simulink model "LoadFlow58BusNetwork_2024"  (R2024a)
settings: Solver=FixedStepDiscrete  StartTime=0.0  StopTime=4.5  FixedStep=75e-6  RelTol=1e-3  EnableMultiTasking=on
undefined symbols (not defined in the file): D1, D11, Delta
libraries: spsSeriesRLCBranchLib x41, spsLoadFlowBusLib x29, spsDistributedParametersLineLib x19, spsThreePhaseSeriesRLCLoadLib x15, spsThreePhaseTransformerTwoWindingsLib x13, spsThreePhaseParallelRLCLoadLib x11, spsThreePhaseVIMeasurementLib x11, spsSynchronousMachinepuStandardLib x7, spsExcitationSystemLib x7, spsHydraulicTurbineandGovernorLib x7, spsGenericPowerSystemStabilizerLib x7, spsMultiBandPowerSystemStabilizerLib x7
(part 2 of 5)

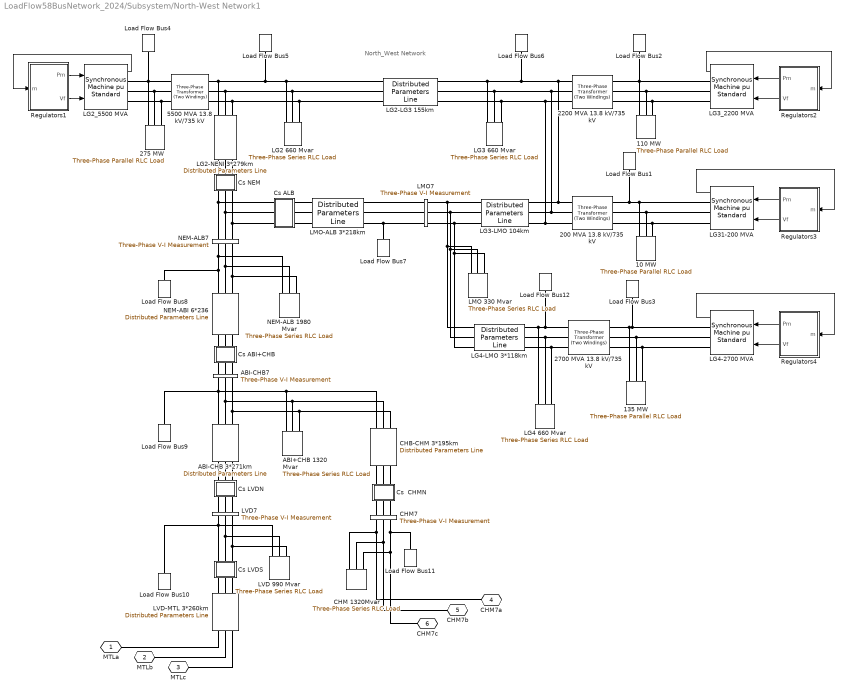
== system LoadFlow58BusNetwork_2024/Subsystem/North-West Network1 ==
  note: North_West Network
  10 MW : spsThreePhaseParallelRLCLoadLib/Three-Phase Parallel RLC Load  LConnTagsString=A|B|C  Configuration=Y (grounded)  NominalVoltage=(13800)*1  Vabc=[1e3 1e3 1e3]  Vabcp=[1e3 1e3 1e3]  NominalFrequency=60  UnbalancedPower=off  ActivePower=10000000  InductivePower=0  CapacitivePower=0  Pabc=[10e3 9e3 11e3]  QLabc=[100 90 110]  QCabc=[100 90 110]  Pabcp=[10e3 9e3 11e3]  QLabcp=[100 90 110]  QCabcp=[100 90 110]  Measurements=None  LoadType=constant PQ
  110 MW : spsThreePhaseParallelRLCLoadLib/Three-Phase Parallel RLC Load  LConnTagsString=A|B|C  Configuration=Y (grounded)  NominalVoltage=(13800)*1  Vabc=[1e3 1e3 1e3]  Vabcp=[1e3 1e3 1e3]  NominalFrequency=60  UnbalancedPower=off  ActivePower=110000000  InductivePower=0  CapacitivePower=0  Pabc=[10e3 9e3 11e3]  QLabc=[100 90 110]  QCabc=[100 90 110]  Pabcp=[10e3 9e3 11e3]  QLabcp=[100 90 110]  QCabcp=[100 90 110]  Measurements=None  LoadType=constant PQ
  135 MW : spsThreePhaseParallelRLCLoadLib/Three-Phase Parallel RLC Load  LConnTagsString=A|B|C  Configuration=Y (grounded)  NominalVoltage=(13800)*1  Vabc=[1e3 1e3 1e3]  Vabcp=[1e3 1e3 1e3]  NominalFrequency=60  UnbalancedPower=off  ActivePower=135000000  InductivePower=0  CapacitivePower=0  Pabc=[10e3 9e3 11e3]  QLabc=[100 90 110]  QCabc=[100 90 110]  Pabcp=[10e3 9e3 11e3]  QLabcp=[100 90 110]  QCabcp=[100 90 110]  Measurements=None  LoadType=constant PQ
  200 MVA 13.8 kV/735 kV : spsThreePhaseTransformerTwoWindingsLib/Three-Phase Transformer (Two Windings)  Winding1Connection=Delta (D1)  Winding2Connection=Yg  CoreType=Three single-phase transformers  SetSaturation=off  Hysteresis=off  DataFile='basic_model'  SetInitialFlux=off  Measurements=None  UNITS=pu  NominalPower=[ 200e6 60 ]  Winding1="[ 13.8e3 0.002  0.0]"  Winding2=[ 735e3 0.002 0.12]  Rm=500  Lm=500  L0=0.5  Saturation="[ 0,0  ;  0.005,1.2  ;  1.0,1.4 ]"  InitialFluxes=[ 0.8 , -0.8 , 0.7 ]  BreakLoop=off  DiscreteSolver=Trapezoidal iterative  DataType=off  TransfoNumber=0
  2200 MVA 13.8 kV/735 kV : spsThreePhaseTransformerTwoWindingsLib/Three-Phase Transformer (Two Windings)  Winding1Connection=Delta (D1)  Winding2Connection=Yg  CoreType=Three single-phase transformers  SetSaturation=off  Hysteresis=off  DataFile='basic_model'  SetInitialFlux=off  Measurements=None  UNITS=pu  NominalPower=[ 2200e6 60 ]  Winding1="[ 13.8e3 0.002  0.0]"  Winding2=[ 735e3 0.002 0.12]  Rm=500  Lm=500  L0=0.5  Saturation="[ 0,0  ;  0.005,1.2  ;  1.0,1.4 ]"  InitialFluxes=[ 0.8 , -0.8 , 0.7 ]  BreakLoop=off  DiscreteSolver=Trapezoidal iterative  DataType=off  TransfoNumber=0
  2700 MVA 13.8 kV/735 kV : spsThreePhaseTransformerTwoWindingsLib/Three-Phase Transformer (Two Windings)  Winding1Connection=Delta (D1)  Winding2Connection=Yg  CoreType=Three single-phase transformers  SetSaturation=off  Hysteresis=off  DataFile='basic_model'  SetInitialFlux=off  Measurements=None  UNITS=pu  NominalPower=[ 2700e6 60 ]  Winding1="[ 13.8e3 0.002  0.0]"  Winding2=[ 735e3 0.002 0.12]  Rm=500  Lm=500  L0=0.5  Saturation="[ 0,0  ;  0.005,1.2  ;  1.0,1.4 ]"  InitialFluxes=[ 0.8 , -0.8 , 0.7 ]  BreakLoop=off  DiscreteSolver=Trapezoidal iterative  DataType=off  TransfoNumber=0
  275 MW : spsThreePhaseParallelRLCLoadLib/Three-Phase Parallel RLC Load  LConnTagsString=A|B|C  Configuration=Y (grounded)  NominalVoltage=(13800)*1  Vabc=[1e3 1e3 1e3]  Vabcp=[1e3 1e3 1e3]  NominalFrequency=60  UnbalancedPower=off  ActivePower=275000000  InductivePower=0  CapacitivePower=0  Pabc=[10e3 9e3 11e3]  QLabc=[100 90 110]  QCabc=[100 90 110]  Pabcp=[10e3 9e3 11e3]  QLabcp=[100 90 110]  QCabcp=[100 90 110]  Measurements=None  LoadType=constant PQ
  5500 MVA 13.8 kV/735 kV : spsThreePhaseTransformerTwoWindingsLib/Three-Phase Transformer (Two Windings)  Winding1Connection=Delta (D1)  Winding2Connection=Yg  CoreType=Three single-phase transformers  SetSaturation=off  Hysteresis=off  DataFile='basic_model'  SetInitialFlux=off  Measurements=None  UNITS=pu  NominalPower=[ 5500e6 60 ]  Winding1="[ 13.8e3 0.002  0.0]"  Winding2=[ 735e3 0.002 0.12]  Rm=500  Lm=500  L0=0.5  Saturation="[ 0,0  ;  0.005,1.2  ;  1.0,1.4 ]"  InitialFluxes=[ 0.8 , -0.8 , 0.7 ]  BreakLoop=off  DiscreteSolver=Trapezoidal iterative  DataType=off  TransfoNumber=0
  ABI+CHB 1320 Mvar : spsThreePhaseSeriesRLCLoadLib/Three-Phase Series RLC Load  LConnTagsString=A|B|C  Configuration=Y (grounded)  NominalVoltage=735e3  Vabc=[1e3 1e3 1e3]  Vabcp=[1e3 1e3 1e3]  NominalFrequency=60  UnbalancedPower=off  ActivePower=4400000  InductivePower=1320e6  CapacitivePower=0  Pabc=[10e3 9e3 11e3]  QLabc=[100 90 110]  QCabc=[100 90 110]  Pabcp=[10e3 9e3 11e3]  QLabcp=[100 90 110]  QCabcp=[100 90 110]  Measurements=None  LoadType=constant Z
  ABI-CHB 3*271km : spsDistributedParametersLineLib/Distributed Parameters Line  Phases=3  Length=271  Frequency=60  Resistance="[0.01273  0.3864]/3"  Inductance="[0.9337e-3  4.1264e-3]/3"  Capacitance=[12.74e-9 7.751e-9]*3  x1=[-0.001575 2.74195871490081e-08 -34814.2579740979 -747194.944177986;-0.0015 2.75338105936338e-08 -13676.7298713989 -747880.497252652;-0.001425 2.76260239313523e-08 7471.73119989829 -747968.20610077;-0.00135 2.76961534482325e-08 28614.2194835957 -747458.000609228;-0.001275 2.77441430838115e-08 49733.83399805 -746350.28862849;-0.0012 2.77699544759089e-08 70813.6920465595 -744645.955646565;-0.001125 2.77735669912929e-08 91836.9427131329 -742346.364081161;-0.00105 2.77549777421738e-08 112786.780332854 -739453.352190591;-0.000975 2.7714201588513e-08 133646.457926072 -735969.232604295;-0.0009 2.76512711261439e-08 154399.300585684 -731896.790474162;-0.000825 2.75662366607152e-08 175028.718806795 -727239.281248121;-0.00075 2.74591661674775e-08 195518.221748122 -722000.428067784;-0.000675 2.73301452369448e-08 215851.430414513 -716184.418792227;-0.0006 2.7179277006475e-08 236012.090750068 -709795.902650276;-0.000525 2.7006682077823e-08 255984.086631383 -702839.986523989;-0.00045 2.68124984207341e-08 275751.452750533 -695322.230866286;-0.000375 2.65968812626527e-08 295298.387377493 -687248.645256015;-0.0003 2.63600029646359e-08 314609.264991801 -678625.683593984;-0.000225 2.61020528835707e-08 333668.648773357 -669460.238943809;-0.00015 2.58232372208051e-08 352461.302942385 -659759.638021708;-7.5e-05 2.55237788573141e-08 370972.20493868 -649531.635339633]  x2=[-0.001575 6.23609378461212e-08 -284619.341076135 -691578.758256646;-0.0015 6.2553714796313e-08 -264954.255311327 -699348.68385095;-0.001425 6.26964872640005e-08 -245077.369168759 -706559.560807776;-0.00135 6.27891411190576e-08 -225004.571927087 -713205.624862417;-0.001275 6.28316022954102e-08 -204751.909473303 -719281.563252954;-0.0012 6.28238368502436e-08 -184335.571475894 -724782.518967204;-0.001125 6.27658509911358e-08 -163771.878443077 -729704.094625337;-0.00105 6.26576910710955e-08 -143077.268676425 -734042.355995072;-0.000975 6.24994435515077e-08 -122268.28513035 -737793.83513665;-0.0009 6.22912349330185e-08 -101361.562187909 -740955.533175044;-0.000825 6.20332316544116e-08 -80373.8123635385 -743524.922697218;-0.00075 6.17256399595605e-08 -59321.8129433254 -745499.9497725;-0.000675 6.13687057325596e-08 -38222.3925734996 -746879.035594466;-0.0006 6.09627143011688e-08 -17092.4178078727 -747661.07774301;-0.000525 6.05079902087265e-08 4051.22037502704 -747845.451065604;-0.00045 6.00048969547146e-08 25191.6200743447 -747432.008177036;-0.000375 5.94538367041829e-08 46311.8819780197 -746421.079577224;-0.0003 5.8855249966264e-08 67395.122871837 -744813.473387024;-0.000225 5.82096152420376e-08 88424.4891356105 -742610.474702226;-0.00015 5.75174486420237e-08 109383.170215709 -739813.844566273;-7.5e-05 5.67793034736118e-08 130254.412063156 -736425.818562504]  x3=[-0.001575 1.26976511809194e-10 -354.964030660685 -109.750554353959;-0.0015 1.34931646331752e-10 -351.719210477034 -119.741131838097;-0.001425 1.42778918560755e-10 -348.193231338013 -129.635990093544;-0.00135 1.50512055506852e-10 -344.388911857396 -139.427219322008;-0.001275 1.58124875418688e-10 -340.309293149966 -149.106992564654;-0.0012 1.65611292724507e-10 -335.957636400499 -158.667571958857;-0.001125 1.72965322896859e-10 -331.337420256818 -168.101314923731;-0.00105 1.80181087236545e-10 -326.452338049017 -177.400680269492;-0.000975 1.87252817571958e-10 -321.306294837067 -186.558234225766;-0.0009 1.94174860870068e-10 -315.903404289175 -195.566656384037;-0.000825 2.00941683755373e-10 -310.247985393379 -204.418745549465;-0.00075 2.07547876933195e-10 -304.344559005013 -213.107425497413;-0.000675 2.13988159513786e-10 -298.197844232806 -221.625750630071;-0.0006 2.2025738323379e-10 -291.812754666499 -229.966911528663;-0.000525 2.26350536571688e-10 -285.194394448997 -238.12424039679;-0.00045 2.3226274875393e-10 -278.348054196193 -246.091216390567;-0.000375 2.37989293648557e-10 -271.279206767732 -253.861470831284;-0.0003 2.435255935432e-10 -263.993502892093 -261.428792296429;-0.000225 2.48867222804431e-10 -256.496766649477 -268.787131585007;-0.00015 2.54009911415548e-10 -248.794990816134 -275.930606553176;-7.5e-05 2.58949548389962e-10 -240.894332073824 -282.853506816347]  x4=[-0.001575 1.8709121084467e-10 -5971.27343085291 -15054.8004559038;-0.0015 1.83115936519456e-10 -5543.2793985662 -15217.5948036282;-0.001425 1.78994282116356e-10 -5110.85415354329 -15368.2244389036;-0.00135 1.74729542422837e-10 -4674.34336990873 -15506.5689507043;-0.001275 1.70325126606556e-10 -4234.09598770412 -15632.5177485442;-0.0012 1.65784555490128e-10 -3790.46393395078 -15745.9701508815;-0.001125 1.6111145873663e-10 -3343.80184132468 -15846.8354656016;-0.00105 1.56309571948106e-10 -2894.46676466851 -15935.0330625152;-0.000975 1.51382733679383e-10 -2442.81789556749 -16010.4924378129;-0.0009 1.46334882369591e-10 -1989.21627521713 -16073.1532704244;-0.000825 1.41170053193831e-10 -1534.02450581238 -16122.9654702391;-0.00075 1.35892374837522e-10 -1077.60646068905 -16159.8892181466;-0.000675 1.3050606619599e-10 -620.326993448974 -16183.8949978676;-0.0006 1.25015433001952e-10 -162.551646301657 -16194.9636195492;-0.000525 1.19424864383572e-10 295.353642144589 -16193.0862351047;-0.00045 1.13738829355866e-10 753.022829408368 -16178.2643452863;-0.000375 1.07961873248235e-10 1210.09006174395 -16150.509798486;-0.0003 1.02098614071001e-10 1666.18996659918 -16109.8447812639;-0.000225 9.61537388238404e-11 2120.95794468867 -16056.3018006126;-0.00015 9.01319997490654e-11 2574.03046144892 -15989.9236579715;-7.5e-05 8.40382105327568e-11 3025.04533764227 -15910.7634150122]  x5=0.00153261764655846  V1=ones(3,3)  V2=ones(3,3)  I1=ones(3,3)  I2=ones(3,3)  nHarmo=1  Measurements=None  Decoupling=on  VsMag0=[610743.955114576 610743.501375021 610743.958218031]  VrMag0=[610622.360478061 610622.247686743 610622.214003654]  VsAngle0=[1.35232982185966 -118.647645266061 121.352379141747]  VrAngle0=[-18.3496130787512 -138.34962283858 101.650391206841]  IsMag0=[305.299965909112 305.301188713068 305.286778308149]  IrMag0=[13308.3117169381 13308.3164139128 13308.3246262143]  IsAngle0=[-68.7963830004266 171.200626740019 51.2019231191185]  IrAngle0=[-17.6151010152143 -137.615048514484 102.384907722659]
      settings: AttributesFormatString=\n  LibrarySourceBlock=sps_lib/Power Grid Elements/Distributed Parameters Line
  ABI-CHB7 : spsThreePhaseVIMeasurementLib/Three-Phase V-I Measurement  VoltageMeasurement=no  SetLabelV=on  LabelV=Vabc_ABI7  Vpu=on  VpuLL=off  CurrentMeasurement=no  SetLabelI=off  LabelI=A1  Ipu=off  Pbase=100e6  Vbase=500e3  OutputType=Magnitude  PhasorSimulation=off  PSBequivalent=0
  CHB-CHM 3*195km : spsDistributedParametersLineLib/Distributed Parameters Line  Phases=3  Length=195  Frequency=60  Resistance="[0.01273  0.3864]/3"  Inductance="[0.9337e-3  4.1264e-3]/3"  Capacitance=[12.74e-9 7.751e-9]*3  x1=[-0.001125 2.77735669912929e-08 0 0;-0.00105 2.77549777421738e-08 0 0;-0.000975 2.7714201588513e-08 0 0;-0.0009 2.76512711261439e-08 0 0;-0.000825 2.75662366607152e-08 0 0;-0.00075 2.74591661674775e-08 0 0;-0.000675 2.73301452369448e-08 215851.430414513 -716184.418792227;-0.0006 2.7179277006475e-08 236012.090750068 -709795.902650276;-0.000525 2.7006682077823e-08 255984.086631383 -702839.986523989;-0.00045 2.68124984207341e-08 275751.452750533 -695322.230866286;-0.000375 2.65968812626527e-08 295298.387377493 -687248.645256015;-0.0003 2.63600029646359e-08 314609.264991801 -678625.683593984;-0.000225 2.61020528835707e-08 333668.648773357 -669460.238943809;-0.00015 2.58232372208051e-08 352461.302942385 -659759.638021708;-7.5e-05 2.55237788573141e-08 370972.20493868 -649531.635339633]  x2=[-0.001125 1.8633658273501e-08 0 0;-0.00105 1.85751782956152e-08 0 0;-0.000975 1.85018496044097e-08 0 0;-0.0009 1.84137308177181e-08 0 0;-0.000825 1.83108923763505e-08 0 0;-0.00075 1.81934164877832e-08 0 0;-0.000675 1.80613970604442e-08 127559.107191249 -726636.134488392;-0.0006 1.79149396286437e-08 148050.539525872 -722739.535823059;-0.000525 1.77541612682118e-08 168423.622524447 -718265.190231074;-0.00045 1.75791905029099e-08 188662.070256145 -713216.674435845;-0.000375 1.73901672016907e-08 208749.704415505 -707598.024143653;-0.0003 1.71872424668888e-08 228670.467255134 -701413.730817573;-0.000225 1.69705785134326e-08 248408.434422015 -694668.738087067;-0.00015 1.67403485391713e-08 267947.827687194 -687368.437796123;-7.5e-05 1.64967365864237e-08 287273.027558661 -679518.665693095]  x3=[-0.001125 9.72668879848698e-11 0 0;-0.00105 9.53952801215306e-11 0 0;-0.000975 9.34474147308589e-11 0 0;-0.0009 9.14248489066448e-11 0 0;-0.000825 8.93291994570618e-11 0 0;-0.00075 8.71621416122154e-11 0 0;-0.000675 8.49254076849897e-11 771.180648774793 -4323.83757003386;-0.0006 8.2620785686263e-11 893.110598565608 -4300.30718909123;-0.000525 8.0250117895599e-11 1014.32660940898 -4273.33920837854;-0.00045 7.78152993885573e-11 1134.73178308051 -4242.95518568696;-0.000375 7.53182765217984e-11 1254.22986952662 -4209.17940953933;-0.0003 7.27610453771962e-11 1372.72534380539 -4172.03887977432;-0.000225 7.01456501662009e-11 1490.12348244773 -4131.56328596315;-0.00015 6.74741815957271e-11 1606.33043917785 -4087.78498367622;-7.5e-05 6.47487751968752e-11 1721.25331993257 -4040.73896861855]  x4=[-0.001125 7.65150883626071e-11 0 0;-0.00105 7.9229424141971e-11 0 0;-0.000975 8.18804251319266e-11 0 0;-0.0009 8.44659721628444e-11 0 0;-0.000825 8.69839983879878e-11 0 0;-0.00075 8.94324909357197e-11 0 0;-0.000675 9.18094925185605e-11 979.606952616345 -12037.6056406812;-0.0006 9.41131029978144e-11 1319.52443201669 -12005.1005057401;-0.000525 9.63414809025106e-11 1658.38710377549 -11962.9986771389;-0.00045 9.84928449014474e-11 1995.92408625771 -11911.3338104353;-0.000375 1.00565475227161e-10 2331.86555756403 -11850.1472057331;-0.0003 1.02557715050681e-10 2665.94297122237 -11779.4877746679;-0.000225 1.04467971805976e-10 2997.88927085982 -11699.4120013079;-0.00015 1.06294718463023e-10 3327.43910368338 -11609.9838970011;-7.5e-05 1.08036494748493e-10 3654.32903259898 -11511.2749492057]  x5=0.0011028060556417  V1=ones(3,3)  V2=ones(3,3)  I1=ones(3,3)  I2=ones(3,3)  nHarmo=1  Measurements=None  Decoupling=on  VsMag0=[610743.955114576 610743.501375021 610743.958218031]  VrMag0=[602368.350238963 602368.356498677 602368.322152166]  VsAngle0=[1.35232982185966 -118.647645266061 121.352379141747]  VrAngle0=[-5.46332293594966 -125.463326364548 114.536674834112]  IsMag0=[3602.61669203533 3602.60152789052 3602.59275066803]  IrMag0=[9906.44607872324 9906.45414351771 9906.46948058251]  IsAngle0=[-5.30716137481158 -125.307461802358 114.692897272091]  IrAngle0=[-10.767651097751 -130.767521740259 109.232373186016]
      settings: AttributesFormatString=\n  LibrarySourceBlock=sps_lib/Power Grid Elements/Distributed Parameters Line
  CHM 1320Mvar : spsThreePhaseSeriesRLCLoadLib/Three-Phase Series RLC Load  LConnTagsString=A|B|C  Configuration=Y (grounded)  NominalVoltage=735e3  Vabc=[1e3 1e3 1e3]  Vabcp=[1e3 1e3 1e3]  NominalFrequency=60  UnbalancedPower=off  ActivePower=4400000  InductivePower=1320e6  CapacitivePower=0  Pabc=[10e3 9e3 11e3]  QLabc=[100 90 110]  QCabc=[100 90 110]  Pabcp=[10e3 9e3 11e3]  QLabcp=[100 90 110]  QCabcp=[100 90 110]  Measurements=None  LoadType=constant Z
  CHM7 : spsThreePhaseVIMeasurementLib/Three-Phase V-I Measurement  VoltageMeasurement=no  SetLabelV=on  LabelV=Vabc_CHM7  Vpu=on  VpuLL=off  CurrentMeasurement=no  SetLabelI=off  LabelI=A1  Ipu=off  Pbase=100e6  Vbase=735e3  OutputType=Magnitude  PhasorSimulation=off  PSBequivalent=0
  "Cs  CHMN " : Subsystem  mask{Xc=25/3}
      mask prompts: Xc "Condensator Reactance at  60Hz  (ohm):"
      mask help: Series Compensation
      mask init:
      | Cs=1/Xc/(2*pi*60);
      mask Display: disp('Cs')
  "Cs ABI+CHB " : Subsystem  mask{Xc=25/6}
      mask prompts: Xc "Condensator Reactance at  60Hz  (ohm):"
      mask help: Series Compensation
      mask init:
      | Cs=1/Xc/(2*pi*60);
      mask Display: disp('Cs')
  Cs ALB : Subsystem  mask{Xc=16/3}
      mask prompts: Xc "Reactance @ 60Hz du condensateur (ohm):"
      mask init:
      | Cs=1/Xc/(2*pi*60);
      mask Display: disp('Cs')
  "Cs LVDN " : Subsystem  mask{Xc=34/3}
      mask prompts: Xc "Condensator Reactance at  60Hz  (ohm):"
      mask help: Series Compensation
      mask init:
      | Cs=1/Xc/(2*pi*60);
      mask Display: disp('Cs')
  "Cs LVDS " : Subsystem  mask{Xc=34/3}
      mask prompts: Xc "Condensator Reactance at  60Hz  (ohm):"
      mask help: Series Compensation
      mask init:
      | Cs=1/Xc/(2*pi*60);
      mask Display: disp('Cs')
  "Cs NEM " : Subsystem  mask{Xc=16/3}
      mask prompts: Xc "Condensator Reactance at  60Hz  (ohm):"
      mask help: Series Compensation
      mask init:
      | Cs=1/Xc/(2*pi*60);
      mask Display: disp('Cs')
  LG2 660 Mvar : spsThreePhaseSeriesRLCLoadLib/Three-Phase Series RLC Load  LConnTagsString=A|B|C  Configuration=Y (grounded)  NominalVoltage=735e3  Vabc=[1e3 1e3 1e3]  Vabcp=[1e3 1e3 1e3]  NominalFrequency=60  UnbalancedPower=off  ActivePower=2200000  InductivePower=660e6  CapacitivePower=0  Pabc=[10e3 9e3 11e3]  QLabc=[100 90 110]  QCabc=[100 90 110]  Pabcp=[10e3 9e3 11e3]  QLabcp=[100 90 110]  QCabcp=[100 90 110]  Measurements=None  LoadType=constant Z
  LG2-LG3 155km : spsDistributedParametersLineLib/Distributed Parameters Line  Phases=3  Length=155  Frequency=60  Resistance="[0.01273  0.3864]"  Inductance="[0.9337e-3  4.1264e-3]"  Capacitance=[12.74e-9 7.751e-9]  x1=[-0.0009 5.26292056031291e-10 425726.576739823 -584301.004479567;-0.000825 5.67978956510661e-10 442074.911234249 -572031.872777898;-0.00075 6.09211823302567e-10 458069.857808607 -559305.467549511;-0.000675 6.49957695484177e-10 473698.630347337 -546131.962088026;-0.0006 6.90184001428704e-10 488948.735448799 -532521.887092147;-0.000525 7.29858584842658e-10 503807.98241231 -518486.122247585;-0.00045 7.689497304711e-10 518264.492983202 -504035.887530001;-0.000375 8.07426189450328e-10 532306.710848115 -489182.734235934;-0.0003 8.45257204287745e-10 545923.410872942 -473938.535748865;-0.000225 8.82412533448924e-10 559103.708076025 -458315.478047822;-0.00015 9.18862475532227e-10 571837.066329446 -442326.049966089;-7.5e-05 9.54577893011657e-10 584113.306781444 -425983.033207829]  x2=[-0.0009 -3.22878941571771e-10 428602.512418869 -576982.581433546;-0.000825 -3.66107619303742e-10 444742.801992339 -564635.073573928;-0.00075 -4.09043636206475e-10 460527.57097469 -551836.205075701;-0.000675 -4.51652669885003e-10 475944.201263112 -538596.207158514;-0.0006 -4.93900659329742e-10 490980.369039234 -524925.663674123;-0.000525 -5.35753832144346e-10 505624.054620598 -510835.502645822;-0.00045 -5.77178731542843e-10 519863.552069006 -496336.987532752;-0.000375 -6.18142243094475e-10 533687.478548069 -481441.708226059;-0.0003 -6.58611621194871e-10 547084.783422473 -466161.571784115;-0.000225 -6.98554515242379e-10 560044.757091687 -450508.792914197;-0.00015 -7.37938995498645e-10 572557.039551054 -434495.88420824;-7.5e-05 -7.76733578612755e-10 584611.62867342 -418135.646140457]  x3=[-0.0009 1.17904511962601e-11 1482.81916403298 -2352.9405377954;-0.000825 1.1694023339197e-11 1548.74539245894 -2310.07973089082;-0.00075 1.15882474588011e-11 1613.43357751477 -2265.37228159477;-0.000675 1.14732081106927e-11 1676.8320084551 -2218.85392835817;-0.0006 1.13489972555666e-11 1738.89000554425 -2170.56185724085;-0.000525 1.12157141856799e-11 1799.55796056888 -2120.53467218556;-0.00045 1.10734654454794e-11 1858.787376494 -2068.8123641586;-0.000375 1.09223647464314e-11 1916.53090623074 -2015.43627918161;-0.0003 1.07625328761229e-11 1972.74239048495 -1960.44908528026;-0.000225 1.05940976017056e-11 2027.37689465618 -1903.89473837601;-0.00015 1.04171935677605e-11 2080.39074475772 -1845.81844714847;-7.5e-05 1.02319621886658e-11 2131.74156232896 -1786.26663689625]  x4=[-0.0009 -1.3249126037137e-11 1223.55408119259 -2231.14873574783;-0.000825 -1.31372285408967e-11 1286.14070278673 -2195.66620561445;-0.00075 -1.30148293451671e-11 1347.69920318167 -2158.42849351113;-0.000675 -1.28820262939926e-11 1408.18037345408 -2119.46536669515;-0.0006 -1.27389255481003e-11 1467.53586588183 -2078.80797169395;-0.000525 -1.25856415000369e-11 1525.71823259244 -2036.48880940701;-0.00045 -1.24222966827252e-11 1582.6809634922 -1992.54170912515;-0.000375 -1.22490216715128e-11 1638.37852344556 -1947.00180148792;-0.0003 -1.20659549797925e-11 1692.76638867532 -1899.90549040071;-0.000225 -1.18732429482767e-11 1745.80108235417 -1851.29042393401;-0.00015 -1.16710396280147e-11 1797.44020935943 -1801.1954642281;-7.5e-05 -1.1459506657247e-11 1847.64249016309 -1749.66065642731]  x5=0.000876589428843401  V1=ones(3,3)  V2=ones(3,3)  I1=ones(3,3)  I2=ones(3,3)  nHarmo=1  Measurements=None  Decoupling=on  VsMag0=[590283.05661746 590282.243891859 590283.870916855]  VrMag0=[586861.315379363 586860.569064535 586862.120536166]  VsAngle0=[25.5173905041478 -94.4824726828172 145.517527228798]  VrAngle0=[26.0462334057268 -93.9536337576198 146.04636292545]  IsMag0=[2279.13376434155 2279.1300076277 2279.13554694054]  IrMag0=[2085.26033535345 2085.25824212135 2085.26456016745]  IsAngle0=[21.6590596698395 -98.3408340586434 141.659194593862]  IrAngle0=[18.1802070278314 -101.819625724334 138.180340460898]
      settings: AttributesFormatString=\n  LibrarySourceBlock=sps_lib/Power Grid Elements/Distributed Parameters Line
  LG2-NENI 3*279km : spsDistributedParametersLineLib/Distributed Parameters Line  Phases=3  Length=279  Frequency=60  Resistance="[0.01273  0.3864]/3"  Inductance="[0.9337e-3  4.1264e-3]/3"  Capacitance=[12.74e-9 7.751e-9]*3  x1=[-0.00165 9.19274009253425e-11 245808.02060678 -679875.080306758;-0.001575 1.36275318057477e-10 264930.184927445 -672654.157661315;-0.0015 1.80514298785439e-10 283840.568111848 -664895.525574191;-0.001425 2.24608979144913e-10 302524.053489008 -656605.386177166;-0.00135 2.68524110523091e-10 320965.705766582 -647790.36648083;-0.001275 3.12224587835874e-10 339150.782969907 -638457.513077055;-0.0012 3.55675477590337e-10 357064.748226506 -628614.286506053;-0.001125 3.98842045810032e-10 374693.281386647 -618268.555292539;-0.00105 4.41689785800794e-10 392022.290470647 -607428.589655751;-0.000975 4.84184445734868e-10 409037.922933787 -596103.05489836;-0.0009 5.26292056031291e-10 425726.576739823 -584301.004479567;-0.000825 5.67978956510661e-10 442074.911234249 -572031.872777898;-0.00075 6.09211823302567e-10 458069.857808607 -559305.467549511;-0.000675 6.49957695484177e-10 473698.630347337 -546131.962088026;-0.0006 6.90184001428704e-10 488948.735448799 -532521.887092147;-0.000525 7.29858584842658e-10 503807.98241231 -518486.122247585;-0.00045 7.689497304711e-10 518264.492983202 -504035.887530001;-0.000375 8.07426189450328e-10 532306.710848115 -489182.734235934;-0.0003 8.45257204287745e-10 545923.410872942 -473938.535748865;-0.000225 8.82412533448924e-10 559103.708076025 -458315.478047822;-0.00015 9.18862475532227e-10 571837.066329446 -442326.049966089;-7.5e-05 9.54577893011657e-10 584113.306781444 -425983.033207829]  x2=[-0.00165 1.5726717321095e-08 25617.0786733605 -737924.87218898;-0.001575 1.58063509389723e-08 46468.3767746725 -736905.697758462;-0.0015 1.58733492017542e-08 67282.5287665809 -735297.452188191;-0.001425 1.59276585520547e-08 88042.8961344504 -733101.42108507;-0.00135 1.59692355758099e-08 108732.883358252 -730319.359922761;-0.001275 1.59980470369834e-08 129335.951178765 -726953.49263839;-0.0012 1.60140699041338e-08 149835.629818813 -723006.509854766;-0.001125 1.60172913688263e-08 170215.532148945 -718481.566729534;-0.00105 1.60077088558714e-08 190459.366787063 -713382.280432996;-0.000975 1.59853300253833e-08 210550.951121497 -707712.727256594;-0.0009 1.59501727666566e-08 230474.224247142 -701477.439354391;-0.000825 1.59022651838661e-08 250213.259804298 -694681.401120133;-0.00075 1.58416455736004e-08 269752.278709957 -687330.045202802;-0.000675 1.57683623942485e-08 289075.661771364 -679429.248163837;-0.0006 1.56824742272626e-08 308167.962171757 -670985.325779507;-0.000525 1.55840497303294e-08 327013.917818318 -662005.027992168;-0.00045 1.54731675824857e-08 345598.463542456 -652495.533514469;-0.000375 1.5349916421224e-08 363906.743142671 -642464.444090795;-0.0003 1.52143947716367e-08 381924.121260378 -631919.77842055;-0.000225 1.50667109676571e-08 399636.195079185 -620869.965748133;-0.00015 1.49069830654583e-08 417028.805838284 -609323.839124725;-7.5e-05 1.47353387490815e-08 434088.050150751 -597290.628347289]  x3=[-0.00165 1.04189262880126e-11 -714.300687613131 -1196.52974167799;-0.001575 1.34208600366926e-11 -680.1882934104 -1216.24398928582;-0.0015 1.64120653552053e-11 -645.532167093147 -1234.98599005777;-0.001425 1.93901511197861e-11 -610.360012238492 -1252.74076192519;-0.00135 2.23527366942409e-11 -574.699944928875 -1269.4941119951;-0.001275 2.52974538329908e-11 -538.580471276486 -1285.23264789579;-0.0012 2.82219485742105e-11 -502.030464635916 -1299.94378848248;-0.001125 3.11238831215504e-11 -465.07914252324 -1313.61577389445;-0.00105 3.40009377129342e-11 -427.756043259981 -1326.23767495578;-0.000975 3.68508124749421e-11 -390.091002360626 -1337.79940191186;-0.0009 3.96712292612939e-11 -352.114128682577 -1348.29171249507;-0.000825 4.24599334739644e-11 -313.855780357586 -1357.70621931286;-0.00075 4.52146958654745e-11 -275.346540523931 -1366.03539655254;-0.000675 4.79333143209179e-11 -236.617192878725 -1373.27258599726;-0.0006 5.06136156182974e-11 -197.698697069896 -1379.4120023485;-0.000525 5.32534571657659e-11 -158.622163947521 -1384.44873785078;-0.00045 5.58507287143813e-11 -119.418830694287 -1388.3787662148;-0.000375 5.84033540450072e-11 -80.1200358549647 -1391.19894583601;-0.0003 6.09092926280109e-11 -40.757194284858 -1392.90702230598;-0.000225 6.33665412544312e-11 -1.36177203724593 -1393.50163021451;-0.00015 6.57731356373132e-11 38.0347387900969 -1392.98229424114;-7.5e-05 6.81271519819295e-11 77.4008452292019 -1391.34942953509]  x4=[-0.00165 3.88189081128881e-11 829.758142041827 -14907.5065102223;-0.001575 3.67400015497132e-11 1250.86903709512 -14878.0908857482;-0.0015 3.46317255914403e-11 1670.9800065791 -14836.7819430624;-0.001425 3.24957655616129e-11 2089.75522021268 -14783.6127039017;-0.00135 3.03338289139973e-11 2506.85991549754 -14718.6256709424;-0.001275 2.81476438676711e-11 2921.96066532219 -14641.8727938242;-0.0012 2.59389580255104e-11 3334.72564449849 -14553.4154276229;-0.001125 2.37095369771835e-11 3744.82489501758 -14453.3242838034;-0.00105 2.14611628877652e-11 4151.93058981335 -14341.6793736947;-0.000975 1.91956330731011e-11 4555.71729482228 -14218.5699445297;-0.0009 1.69147585630615e-11 4955.86222913054 -14084.0944081025;-0.000825 1.4620362653831e-11 5352.04552300007 -13938.3602620993;-0.00075 1.23142794503941e-11 5743.95047356756 -13781.4840041667;-0.000675 9.99835240037937e-12 6131.26379801187 -13613.5910387849;-0.0006 7.67443282043569e-12 6513.67588398753 -13434.8155770217;-0.000525 5.3443784163181e-12 6890.88103712411 -13245.3005292457;-0.00045 3.01005179786624e-12 7262.57772539363 -13045.1973908866;-0.000375 6.73318990062507e-13 7628.46882015064 -12834.6661213313;-0.0003 -1.66395205863976e-12 7988.2618336523 -12613.8750160557;-0.000225 -3.99989296952567e-12 8341.66915286865 -12383.000572091;-0.00015 -6.33263642717216e-12 8688.40826939601 -12142.2273469353;-7.5e-05 -8.66031767215134e-12 9028.20200528992 -11891.7478110207]  x5=0.00157786097191812  V1=ones(3,3)  V2=ones(3,3)  I1=ones(3,3)  I2=ones(3,3)  nHarmo=1  Measurements=None  Decoupling=on  VsMag0=[590283.05661746 590282.243891859 590283.870916855]  VrMag0=[602875.980203833 602875.441014975 602876.102194659]  VsAngle0=[25.5173905041478 -94.4824726828172 145.517527228798]  VrAngle0=[7.62822080532469 -112.371736222201 127.628286669386]  IsMag0=[1145.30812027487 1145.28643710013 1145.27794996265]  IrMag0=[12270.9673380103 12270.9820903548 12270.9983548869]  IsAngle0=[-25.195118488194 -145.196235040868 94.8052626724972]  IrAngle0=[8.82574494857689 -111.174127591583 128.825749025244]
      settings: AttributesFormatString=\n  LibrarySourceBlock=sps_lib/Power Grid Elements/Distributed Parameters Line
  LG2_5500 MVA : spsSynchronousMachinepuStandardLib/Synchronous Machine pu Standard  PresetModel=No  MechanicalLoad=Mechanical power Pm  ShowDetailedParameters=on  RotorType=Salient-pole  Units=per unit standard parameters  MeasurementBus=off  NominalParameters="[5500E6  13800   60 ]"  Reactances1=[ 31 32 33 34 35 36 37 ]  Reactances2=[ 1.305, 0.296, 0.252, 0.474, 0.243, 0.18 ]  dAxisTimeConstants=Short-circuit  qAxisTimeConstants=Open-circuit  TimeConstants1=[]  TimeConstants2=[]  TimeConstants3=[]  TimeConstants4=[]  TimeConstants5=[ 1.01, 0.053, 0.1 ]  TimeConstants6=[]  TimeConstants7=[]  TimeConstants8=[]  StatorResistance=2.8544e-3  Mechanical="[ 4.1  0  32]"  PolePairs=32  InitialConditions=[0 -65.2434 0.985682 0.985682 0.985682 -1.22427 -121.224 118.776 1.47412]  SetSaturation=off  Saturation=[0.6404,0.7127,0.8441,0.9214,0.9956,1.082,1.19,1.316,1.457;0.7,0.7698,0.8872,0.9466,0.9969,1.046,1.1,1.151,1.201]  LoadFlowParameters=[2 4000000000 0 0 0]  TsPowergui=0  TsBlock=-1  IterativeModel=Trapezoidal non iterative  IterativeDiscreteModel=Trapezoidal non iterative  BusType=swing  Pref=0  Qref=0  Qmin=-Inf  Qmax=Inf  PLF=0  QLF=0
  LG3 660 Mvar : spsThreePhaseSeriesRLCLoadLib/Three-Phase Series RLC Load  LConnTagsString=A|B|C  Configuration=Y (grounded)  NominalVoltage=735e3  Vabc=[1e3 1e3 1e3]  Vabcp=[1e3 1e3 1e3]  NominalFrequency=60  UnbalancedPower=off  ActivePower=2200000  InductivePower=660e6  CapacitivePower=0  Pabc=[10e3 9e3 11e3]  QLabc=[100 90 110]  QCabc=[100 90 110]  Pabcp=[10e3 9e3 11e3]  QLabcp=[100 90 110]  QCabcp=[100 90 110]  Measurements=None  LoadType=constant Z
  LG3-LMO 104km : spsDistributedParametersLineLib/Distributed Parameters Line  Phases=3  Length=104  Frequency=60  Resistance="[0.01273  0.3864]"  Inductance="[0.9337e-3  4.1264e-3]"  Capacitance=[12.74e-9 7.751e-9]  x1=[-0.0006 -4.93900659329742e-10 0 0;-0.000525 -5.35753832144346e-10 0 0;-0.00045 -5.77178731542843e-10 0 0;-0.000375 -6.18142243094475e-10 533687.478548069 -481441.708226059;-0.0003 -6.58611621194871e-10 547084.783422473 -466161.571784115;-0.000225 -6.98554515242379e-10 560044.757091687 -450508.792914197;-0.00015 -7.37938995498645e-10 572557.039551054 -434495.88420824;-7.5e-05 -7.76733578612755e-10 584611.62867342 -418135.646140457]  x2=[-0.0006 4.47690415711637e-09 0 0;-0.000525 4.40208256148467e-09 0 0;-0.00045 4.32374200840744e-09 0 0;-0.000375 4.24194512212416e-09 480200.396912812 -552194.743514741;-0.0003 4.15675728981419e-09 495619.31477365 -538398.460516366;-0.000225 4.06824660932726e-09 510642.042137489 -524171.790026426;-0.00015 3.9764838347471e-09 525256.570065928 -509526.104627636;-7.5e-05 3.88154231983168e-09 539451.215928951 -494473.111856818]  x3=[-0.0006 1.21767265789831e-11 0 0;-0.000525 1.29310646676612e-11 0 0;-0.00045 1.36750658610958e-11 0 0;-0.000375 1.44081354161167e-11 -139.986222681512 -514.515779236232;-0.0003 1.51296873281377e-11 -125.384058316439 -518.267255559751;-0.000225 1.58391447996006e-11 -110.681663853589 -521.604436968931;-0.00015 1.65359407010578e-11 -95.8907921621402 -524.524655772014;-7.5e-05 1.72195180245269e-11 -81.0232668386155 -527.025577590769]  x4=[-0.0006 -5.58819950672655e-12 0 0;-0.000525 -6.40517588641985e-12 0 0;-0.00045 -7.21703206651204e-12 0 0;-0.000375 -8.02311906159454e-12 3613.50960647484 -3542.58660366458;-0.0003 -8.82279249805705e-12 3712.21557844751 -3439.01470479837;-0.000225 -9.61541312918986e-12 3807.95406208557 -3332.69371019582;-0.00015 -1.04003473461879e-11 3900.64852551005 -3223.70861123327;-7.5e-05 -1.11769676846481e-11 3990.22487018516 -3112.1465289313]  x5=0.000588163229675572  V1=ones(3,3)  V2=ones(3,3)  I1=ones(3,3)  I2=ones(3,3)  nHarmo=1  Measurements=None  Decoupling=on  VsMag0=[586861.315379363 586860.569064535 586862.120536166]  VrMag0=[597501.495499378 597500.918482482 597501.873521838]  VsAngle0=[26.0462334057268 -93.9536337576198 146.04636292545]  VrAngle0=[19.110915447076 -100.889010750021 139.111000266933]  IsMag0=[436.451079902186 436.445924432135 436.434679858849]  IrMag0=[4141.87607401795 4141.88820061772 4141.89211373219]  IsAngle0=[-37.1184575596484 -157.120552820003 82.8810809575978]  IrAngle0=[23.6678939917985 -96.3319466522321 143.667828394017]
      settings: AttributesFormatString=\n  LibrarySourceBlock=sps_lib/Power Grid Elements/Distributed Parameters Line
  LG31-200 MVA : spsSynchronousMachinepuStandardLib/Synchronous Machine pu Standard  PresetModel=No  MechanicalLoad=Mechanical power Pm  ShowDetailedParameters=on  RotorType=Salient-pole  Units=per unit standard parameters  MeasurementBus=off  NominalParameters="[200E6  13800   60 ]"  Reactances1=[ 31 32 33 34 35 36 37 ]  Reactances2=[ 1.305, 0.296, 0.252, 0.474, 0.243, 0.18 ]  dAxisTimeConstants=Short-circuit  qAxisTimeConstants=Open-circuit  TimeConstants1=[]  TimeConstants2=[]  TimeConstants3=[]  TimeConstants4=[]  TimeConstants5=[ 1.01, 0.053, 0.1 ]  TimeConstants6=[]  TimeConstants7=[]  TimeConstants8=[]  StatorResistance=2.8544e-3  Mechanical="[ 3.2  0  32]"  PolePairs=32  InitialConditions=[0 -67.6291 0.902477 0.902477 0.902477 -4.2812 -124.281 115.719 1.45511]  SetSaturation=off  Saturation=[0.6404,0.7127,0.8441,0.9214,0.9956,1.082,1.19,1.316,1.457;0.7,0.7698,0.8872,0.9466,0.9969,1.046,1.1,1.151,1.201]  LoadFlowParameters=[1 180000000 0 0 0]  TsPowergui=0  TsBlock=-1  IterativeModel=Trapezoidal non iterative  IterativeDiscreteModel=Trapezoidal non iterative  BusType=PV  Pref=180000000  Qref=0  Qmin=-Inf  Qmax=Inf  PLF=0  QLF=0
  LG3_2200 MVA : spsSynchronousMachinepuStandardLib/Synchronous Machine pu Standard  PresetModel=No  MechanicalLoad=Mechanical power Pm  ShowDetailedParameters=on  RotorType=Salient-pole  Units=per unit standard parameters  MeasurementBus=off  NominalParameters="[2200E6  13800   60 ]"  Reactances1=[ 31 32 33 34 35 36 37 ]  Reactances2=[ 1.305, 0.296, 0.252, 0.474, 0.243, 0.18 ]  dAxisTimeConstants=Short-circuit  qAxisTimeConstants=Open-circuit  TimeConstants1=[]  TimeConstants2=[]  TimeConstants3=[]  TimeConstants4=[]  TimeConstants5=[ 1.01, 0.053, 0.1 ]  TimeConstants6=[]  TimeConstants7=[]  TimeConstants8=[]  StatorResistance=2.8544e-3  Mechanical="[ 3.2  0  32]"  PolePairs=32  InitialConditions=[0 -70.0065 0.820496 0.820496 0.820496 -4.90643 -124.906 115.094 1.38903]  SetSaturation=off  Saturation=[0.6404,0.7127,0.8441,0.9214,0.9956,1.082,1.19,1.316,1.457;0.7,0.7698,0.8872,0.9466,0.9969,1.046,1.1,1.151,1.201]  LoadFlowParameters=[1 1800000000 0 0 0]  TsPowergui=0  TsBlock=-1  IterativeModel=Trapezoidal non iterative  IterativeDiscreteModel=Trapezoidal non iterative  BusType=PV  Pref=1800000000  Qref=0  Qmin=-Inf  Qmax=Inf  PLF=0  QLF=0
  LG4 660 Mvar : spsThreePhaseSeriesRLCLoadLib/Three-Phase Series RLC Load  LConnTagsString=A|B|C  Configuration=Y (grounded)  NominalVoltage=735e3  Vabc=[1e3 1e3 1e3]  Vabcp=[1e3 1e3 1e3]  NominalFrequency=60  UnbalancedPower=off  ActivePower=2200000  InductivePower=660e6  CapacitivePower=0  Pabc=[10e3 9e3 11e3]  QLabc=[100 90 110]  QCabc=[100 90 110]  Pabcp=[10e3 9e3 11e3]  QLabcp=[100 90 110]  QCabcp=[100 90 110]  Measurements=None  LoadType=constant Z
  LG4-2700 MVA : spsSynchronousMachinepuStandardLib/Synchronous Machine pu Standard  PresetModel=No  MechanicalLoad=Mechanical power Pm  ShowDetailedParameters=on  RotorType=Salient-pole  Units=per unit standard parameters  MeasurementBus=off  NominalParameters="[2700E6  13800   60 ]"  Reactances1=[ 31 32 33 34 35 36 37 ]  Reactances2=[ 1.305, 0.296, 0.252, 0.474, 0.243, 0.18 ]  dAxisTimeConstants=Short-circuit  qAxisTimeConstants=Open-circuit  TimeConstants1=[]  TimeConstants2=[]  TimeConstants3=[]  TimeConstants4=[]  TimeConstants5=[ 1.01, 0.053, 0.1 ]  TimeConstants6=[]  TimeConstants7=[]  TimeConstants8=[]  StatorResistance=2.8544e-3  Mechanical="[ 3.7  0  32]"  PolePairs=32  InitialConditions=[0 -69.506 0.926038 0.926038 0.926038 -2.40174 -122.402 117.598 1.38766]  SetSaturation=off  Saturation=[0.6404,0.7127,0.8441,0.9214,0.9956,1.082,1.19,1.316,1.457;0.7,0.7698,0.8872,0.9466,0.9969,1.046,1.1,1.151,1.201]  LoadFlowParameters=[1 2500000000 0 0 0]  TsPowergui=0  TsBlock=-1  IterativeModel=Trapezoidal non iterative  IterativeDiscreteModel=Trapezoidal non iterative  BusType=PV  Pref=2500000000  Qref=0  Qmin=-Inf  Qmax=Inf  PLF=0  QLF=0
  LG4-LMO 3*118km : spsDistributedParametersLineLib/Distributed Parameters Line  Phases=3  Length=118  Frequency=60  Resistance="[0.01273  0.3864]/3"  Inductance="[0.9337e-3  4.1264e-3]/3"  Capacitance=[12.74e-9 7.751e-9]*3  x1=[-0.000675 -6.41986049789956e-10 446066.32494244 -570785.422694474;-0.0006 -7.05961385910428e-10 462024.453036365 -557946.706607689;-0.000525 -7.69372387300575e-10 477613.245851744 -544661.976460512;-0.00045 -8.32168364176106e-10 492820.241946116 -530941.85186296;-0.000375 -8.94299118393918e-10 507633.28507948 -516797.300472712;-0.0003 -9.55714983579721e-10 522040.533931801 -502239.62922773;-0.000225 -1.01636686483058e-09 536030.471568784 -487280.475307667;-0.00015 -1.07620627796063e-09 549591.914648337 -471931.796831284;-7.5e-05 -1.13518538825858e-09 562714.022360358 -456205.863297313]  x2=[-0.000675 4.54814698406381e-09 414813.875448584 -602860.773675066;-0.0006 4.47690415711637e-09 431691.28099871 -590892.755025168;-0.000525 4.40208256148467e-09 448223.599143904 -578452.385747865;-0.00045 4.32374200840744e-09 464397.614201994 -565549.610484014;-0.000375 4.24194512212416e-09 480200.396912812 -552194.743514741;-0.0003 4.15675728981419e-09 495619.31477365 -538398.460516366;-0.000225 4.06824660932726e-09 510642.042137489 -524171.790026426;-0.00015 3.9764838347471e-09 525256.570065928 -509526.104627636;-7.5e-05 3.88154231983168e-09 539451.215928951 -494473.111856818]  x3=[-0.000675 2.64276877993109e-11 2040.14143601584 -4504.23210447596;-0.0006 2.84204057532515e-11 2166.66257243623 -4444.75566915095;-0.000525 3.03904048696798e-11 2291.45171194727 -4381.72616415107;-0.00045 3.23361103614441e-11 2414.40910002016 -4315.19397429823;-0.000375 3.42559668613445e-11 2535.4364464002 -4245.21228440701;-0.0003 3.61484396654698e-11 2654.43700367846 -4171.83703676957;-0.000225 3.80120159600162e-11 2771.31564463022 -4095.12688643618;-0.00015 3.98452060306076e-11 2885.97893825822 -4015.14315432731;-7.5e-05 4.16465444531501e-11 2998.33522447994 -3931.94977821462]  x4=[-0.000675 -3.12219621864875e-12 6463.18076750033 -9178.78456746738;-0.0006 -5.6030458971222e-12 6720.08725258103 -8992.3975565774;-0.000525 -8.07941658643496e-12 6971.6218027328 -8798.822160669;-0.00045 -1.05493287137477e-11 7217.58334508485 -8598.21312095185;-0.000375 -1.30108078690969e-11 7457.77526174357 -8390.73080122289;-0.0003 -1.54618863837075e-11 7692.00554696584 -8176.54105967391;-0.000225 -1.79006049029178e-11 7920.08696064549 -7955.81511630711;-0.00015 -2.03250139524572e-11 8141.8371779902 -7728.72941606438;-7.5e-05 -2.27331754968261e-11 8357.07893526912 -7495.46548777997]  x5=0.000667339049054976  V1=ones(3,3)  V2=ones(3,3)  I1=ones(3,3)  I2=ones(3,3)  nHarmo=1  Measurements=None  Decoupling=on  VsMag0=[591479.20702059 591478.775968447 591479.558478787]  VrMag0=[597501.495499378 597500.918482482 597501.873521838]  VsAngle0=[22.587469141169 -97.4124674392069 142.587537012211]  VrAngle0=[19.110915447076 -100.889010750021 139.111000266933]  IsMag0=[4048.55267184938 4048.5552176619 4048.56794769907]  IrMag0=[9191.46117506314 9191.4454305137 9191.45421674865]  IsAngle0=[8.94759792224694 -111.052173248451 128.947681135233]  IrAngle0=[19.7310305258229 -100.268962895626 139.73111881125]
      settings: AttributesFormatString=\n  LibrarySourceBlock=sps_lib/Power Grid Elements/Distributed Parameters Line
  LMO 330 Mvar : spsThreePhaseSeriesRLCLoadLib/Three-Phase Series RLC Load  LConnTagsString=A|B|C  Configuration=Y (grounded)  NominalVoltage=735e3  Vabc=[1e3 1e3 1e3]  Vabcp=[1e3 1e3 1e3]  NominalFrequency=60  UnbalancedPower=off  ActivePower=1100000  InductivePower=330e6  CapacitivePower=0  Pabc=[10e3 9e3 11e3]  QLabc=[100 90 110]  QCabc=[100 90 110]  Pabcp=[10e3 9e3 11e3]  QLabcp=[100 90 110]  QCabcp=[100 90 110]  Measurements=None  LoadType=constant Z
  LMO-ALB 3*218km : spsDistributedParametersLineLib/Distributed Parameters Line  Phases=3  Length=218  Frequency=60  Resistance="[0.01273  0.3864]/3"  Inductance="[0.9337e-3  4.1264e-3]/3"  Capacitance=[12.74e-9 7.751e-9]*3  x1=[-0.001275 4.98304059487512e-09 0 0;-0.0012 4.94222885662431e-09 0 0;-0.001125 4.89746637624415e-09 0 0;-0.00105 4.84878893617657e-09 0 0;-0.000975 4.79623544842236e-09 0 0;-0.0009 4.73984792343556e-09 0 0;-0.000825 4.67967143654086e-09 380078.03336525 -625341.876126298;-0.00075 4.61575409190116e-09 397604.874033289 -614346.874646567;-0.000675 4.54814698406381e-09 414813.875448584 -602860.773675066;-0.0006 4.47690415711637e-09 431691.28099871 -590892.755025168;-0.000525 4.40208256148467e-09 448223.599143904 -578452.385747865;-0.00045 4.32374200840744e-09 464397.614201994 -565549.610484014;-0.000375 4.24194512212416e-09 480200.396912812 -552194.743514741;-0.0003 4.15675728981419e-09 495619.31477365 -538398.460516366;-0.000225 4.06824660932726e-09 510642.042137489 -524171.790026426;-0.00015 3.9764838347471e-09 525256.570065928 -509526.104627636;-7.5e-05 3.88154231983168e-09 539451.215928951 -494473.111856818]  x2=[-0.001275 1.63637606646819e-08 0 0;-0.0012 1.63776052289692e-08 0 0;-0.001125 1.63783577862223e-08 0 0;-0.00105 1.63660177348583e-08 0 0;-0.000975 1.63405949393255e-08 0 0;-0.0009 1.63021097222178e-08 0 0;-0.000825 1.62505928480287e-08 256317.712946226 -689303.964750356;-0.00075 1.61860854985593e-08 275702.267037886 -681782.177055729;-0.000675 1.61086392399978e-08 294866.428955661 -673715.38312038;-0.0006 1.60183159816983e-08 313794.879161737 -665110.031415955;-0.000525 1.59151879266915e-08 332472.486542634 -655973.000928942;-0.00045 1.57993375139666e-08 350884.320504788 -646311.595661709;-0.000375 1.5670857352571e-08 369015.662909841 -636133.538793804;-0.0003 1.55298501475799e-08 386852.019840093 -625446.966508156;-0.000225 1.53764286179956e-08 404379.133184719 -614260.421487141;-0.00015 1.52107154066412e-08 421582.992037485 -602582.846083689;-7.5e-05 1.50328429821226e-08 438449.843896853 -590423.575172904]  x3=[-0.001275 2.94646741323298e-11 0 0;-0.0012 3.21727222447971e-11 0 0;-0.001125 3.48550519753611e-11 0 0;-0.00105 3.75095191106761e-11 0 0;-0.000975 4.0134001710329e-11 0 0;-0.0009 4.27264018030854e-11 0 0;-0.000825 4.52846470639763e-11 504.220647789844 -2691.25110183801;-0.00075 4.78066924708826e-11 580.102277877155 -2675.92034910846;-0.000675 5.02905219392946e-11 655.520183079393 -2658.45050659478;-0.0006 5.27341499339392e-11 730.414075477072 -2638.85553942178;-0.000525 5.5135623055986e-11 804.724086038526 -2617.15111150641;-0.00045 5.74930216045653e-11 878.390812478291 -2593.35457303626;-0.000375 5.98044611113466e-11 951.355366742391 -2567.48494660008;-0.0003 6.20680938469544e-11 1023.55942208254 -2539.56291198143;-0.000225 6.42821102980147e-11 1094.94525968167 -2509.61078962755;-0.00015 6.64447406136519e-11 1165.45581479342 -2477.65252280678;-7.5e-05 6.85542560202813e-11 1235.03472235891 -2443.71365846863]  x4=[-0.001275 5.51779426535561e-11 0 0;-0.0012 5.27942986491076e-11 0 0;-0.001125 5.03684516900989e-11 0 0;-0.00105 4.79023409614722e-11 0 0;-0.000975 4.53979378344113e-11 0 0;-0.0009 4.28572442904574e-11 0 0;-0.000825 4.02822913211554e-11 4425.69676226963 -12765.9262438955;-0.00075 3.76751373045111e-11 4784.82745779817 -12635.7066271861;-0.000675 3.50378663595545e-11 5140.13323546727 -12495.3862199317;-0.0006 3.23725866803274e-11 5491.33006927461 -12345.0771921189;-0.000525 2.96814288506252e-11 5838.13721784474 -12184.8996984847;-0.00045 2.69665441408409e-11 6180.27744884941 -12014.9817824668;-0.000375 2.42301027882724e-11 6517.4772606229 -11835.4592738474;-0.0003 2.1474292262268e-11 6849.46710079498 -11646.475680173;-0.000225 1.87013155155967e-11 7175.98158176706 -11448.182072037;-0.00015 1.59133892234421e-11 7496.75969285887 -11240.7369623156;-7.5e-05 1.31127420114252e-11 7811.54500895647 -11024.3061794557]  x5=0.00123288061605072  V1=ones(3,3)  V2=ones(3,3)  I1=ones(3,3)  I2=ones(3,3)  nHarmo=1  Measurements=None  Decoupling=on  VsMag0=[597501.495499378 597500.918482482 597501.873521838]  VrMag0=[600465.939453866 600465.308790899 600466.091594138]  VsAngle0=[19.110915447076 -100.889010750021 139.111000266933]  VrAngle0=[8.21765611493921 -111.782292378918 128.21773398292]  IsMag0=[2247.12525868903 2247.11361991023 2247.12200887493]  IrMag0=[11088.6272022732 11088.6249727985 11088.6349972336]  IsAngle0=[-1.5682919473383 -121.56821629481 118.432002879357]  IrAngle0=[6.94042447158054 -113.059522369362 126.940461027597]
      settings: AttributesFormatString=\n  LibrarySourceBlock=sps_lib/Power Grid Elements/Distributed Parameters Line
  LMO7 : spsThreePhaseVIMeasurementLib/Three-Phase V-I Measurement  VoltageMeasurement=no  SetLabelV=on  LabelV=Vabc_LMO7  Vpu=on  VpuLL=off  CurrentMeasurement=no  SetLabelI=off  LabelI=A1  Ipu=off  Pbase=100e6  Vbase=735e3  OutputType=Magnitude  PhasorSimulation=off  PSBequivalent=0
  LVD 990 Mvar : spsThreePhaseSeriesRLCLoadLib/Three-Phase Series RLC Load  LConnTagsString=A|B|C  Configuration=Y (grounded)  NominalVoltage=735e3  Vabc=[1e3 1e3 1e3]  Vabcp=[1e3 1e3 1e3]  NominalFrequency=60  UnbalancedPower=off  ActivePower=3300000  InductivePower=990e6  CapacitivePower=0  Pabc=[10e3 9e3 11e3]  QLabc=[100 90 110]  QCabc=[100 90 110]  Pabcp=[10e3 9e3 11e3]  QLabcp=[100 90 110]  QCabcp=[100 90 110]  Measurements=None  LoadType=constant Z
  LVD-MTL 3*260km : spsDistributedParametersLineLib/Distributed Parameters Line  Phases=3  Length=260  Frequency=60  Resistance="[0.01273  0.3864]/3"  Inductance="[0.9337e-3  4.1264e-3]/3"  Capacitance=[12.74e-9 7.751e-9]*3  x1=[-0.0015 5.6813264746397e-08 -89258.2599346366 -744297.731345277;-0.001425 5.69990779357158e-08 -68180.8722481689 -746523.607859738;-0.00135 5.71393269342479e-08 -47048.9818156284 -748152.72482427;-0.001275 5.72338996290898e-08 -25879.4811468982 -749183.779947698;-0.0012 5.72827204202762e-08 -4689.29281690833 -749615.949020333;-0.001125 5.72857502812137e-08 16504.6440620108 -749448.886572829;-0.00105 5.72429867898777e-08 37685.3873809962 -748682.726152351;-0.000975 5.7154464130749e-08 58836.0055779151 -747318.080215817;-0.0009 5.70202530674868e-08 79939.5911721959 -745356.039640308;-0.000825 5.68404608863615e-08 100979.274280411 -742798.172851041;-0.00075 5.66152313104919e-08 121938.2361018 -739646.52456759;-0.000675 5.63447443849548e-08 142799.722362967 -735903.614169371;-0.0006 5.60292163328599e-08 163547.056710987 -731572.433681687;-0.000525 5.56688993825042e-08 184163.654044225 -726656.445383953;-0.00045 5.52640815657449e-08 204633.033770219 -721159.579041994;-0.000375 5.48150864877507e-08 224938.832980008 -715086.228766661;-0.0003 5.43222730683172e-08 245064.819528392 -708441.249501238;-0.000225 5.37860352549515e-08 264994.905009662 -701229.953140479;-0.00015 5.32068017079569e-08 284713.157618426 -693458.104284357;-7.5e-05 5.25850354577684e-08 304203.814885246 -685131.915629935]  x2=[-0.0015 8.73187919700411e-08 -318141.458272 -654659.491566377;-0.001425 8.74847463324816e-08 -299506.698691689 -663391.865921032;-0.00135 8.75807667272655e-08 -280632.518039049 -671593.934968305;-0.001275 8.76067763971582e-08 -261534.00404531 -679259.142099697;-0.0012 8.75627545504276e-08 -242226.423770342 -686381.359865907;-0.001125 8.74487363774646e-08 -222725.211398401 -692954.894875028;-0.00105 8.72648130226518e-08 -203045.955900277 -698974.492343751;-0.000975 8.70111315115053e-08 -183204.388571714 -704435.340297963;-0.0009 8.66878946331434e-08 -163216.370458049 -709333.073419362;-0.000825 8.62953607781809e-08 -143097.879675133 -713663.77653503;-0.00075 8.58338437321758e-08 -122864.998636676 -717423.987747158;-0.000675 8.53037124247929e-08 -102533.901198206 -720610.701200436;-0.0006 8.47053906348883e-08 -82120.8397279397 -723221.369484888;-0.000525 8.40393566517461e-08 -61642.1321148858 -725253.905672232;-0.00045 8.33061428927417e-08 -41114.1487245756 -726706.684984138;-0.000375 8.25063354777356e-08 -20553.2993128425 -727578.546091053;-0.0003 8.16405737605379e-08 23.980091885227 -727868.792040548;-0.000225 8.07095498178186e-08 20601.2403272944 -727577.190814452;-0.00015 7.97140078958725e-08 41162.0322463955 -726703.975514322;-7.5e-05 7.86547438156797e-08 61689.9198667191 -725249.844175111]  x3=[-0.0015 2.53462205062267e-10 326.03461791467 -307.945403568491;-0.001425 2.61732433341848e-10 334.61041759976 -298.604572742158;-0.00135 2.69793436718856e-10 342.918734836732 -289.025041989178;-0.001275 2.77638771350529e-10 350.952928083907 -279.214469039864;-0.0012 2.85262165796401e-10 358.706574930133 -269.180696316124;-0.001125 2.92657526031592e-10 366.173477228754 -258.931744662351;-0.00105 2.99818940318283e-10 373.34766605232 -248.475806933684;-0.000975 3.06740683931468e-10 380.223406464055 -237.821241446761;-0.0009 3.13417223735208e-10 386.795202102275 -226.976565298213;-0.000825 3.19843222605739e-10 393.057799574101 -215.950447556223;-0.00075 3.26013543697883e-10 399.006192654932 -204.75170233061;-0.000675 3.3192325455137e-10 404.635626290355 -193.389281726959;-0.0006 3.37567631033765e-10 409.941600397254 -181.872268690452;-0.000525 3.4294216111687e-10 414.919873461112 -170.209869745092;-0.00045 3.48042548483568e-10 419.566465926613 -158.411407634156;-0.000375 3.52864715962239e-10 423.877663378833 -146.486313867733;-0.0003 3.5740480878598e-10 427.850019512495 -134.444121183321;-0.000225 3.61659197674055e-10 431.480358886883 -122.294455925498;-0.00015 3.65624481733081e-10 434.765779464248 -110.047030350776;-7.5e-05 3.69297491175651e-10 437.703654929648 -97.7116348637683]  x4=[-0.0015 2.62978177232356e-10 -7428.61939570876 -14286.168118044;-0.001425 2.60385231618917e-10 -7021.77252832352 -14490.4696992912;-0.00135 2.5758413803535e-10 -6609.31256341587 -14683.1878207725;-0.001275 2.54577135633007e-10 -6191.5692151709 -14864.1684265701;-0.0012 2.51366628163599e-10 -5768.87642122951 -15033.266843557;-0.001125 2.47955182057676e-10 -5341.57207574375 -15190.3478970458;-0.00105 2.44345524373058e-10 -4909.99775926943 -15335.2860188458;-0.000975 2.40540540614868e-10 -4474.49846571185 -15467.9653476401;-0.0009 2.36543272428904e-10 -4035.42232654289 -15588.2798216033;-0.000825 2.32356915170193e-10 -3593.12033251013 -15696.1332631858;-0.00075 2.27984815348676e-10 -3147.94605306014 -15791.4394559966;-0.000675 2.23430467954053e-10 -2700.25535370053 -15874.1222137234;-0.0006 2.18697513661949e-10 -2250.40611152646 -15944.1154410347;-0.000525 2.13789735923608e-10 -1798.75792913921 -16001.3631864157;-0.00045 2.08711057941462e-10 -1345.67184718532 -16045.8196868944;-0.000375 2.03465539532983e-10 -891.51005574626 -16077.4494046248;-0.0003 1.9805737388533e-10 -436.635604809198 -16096.2270552943;-0.000225 1.92490884203372e-10 18.5878859495995 -16102.1376283364;-0.00015 1.8677052025379e-10 473.796517836773 -16095.1763989293;-7.5e-05 1.80900854808003e-10 928.626404036918 -16075.3489317734]  x5=0.00147040807418893  V1=ones(3,3)  V2=ones(3,3)  I1=ones(3,3)  I2=ones(3,3)  nHarmo=1  Measurements=None  Decoupling=on  VsMag0=[612070.919184254 612070.526870881 612070.832121206]  VrMag0=[594302.518281079 594302.525591473 594302.380387402]  VsAngle0=[-4.43840982431361 -124.43839803227 115.561627875922]  VrAngle0=[-23.5181046799965 -143.51812043764 96.4818868308265]  IsMag0=[368.438417399525 368.422778585175 368.434712933316]  IrMag0=[13227.9520808221 13227.9561692161 13227.9649229582]  IsAngle0=[49.0336389584108 -70.9656221606516 169.036114576079]  IrAngle0=[-25.073891325028 -145.073837319251 94.9261203418354]
      settings: AttributesFormatString=\n  LibrarySourceBlock=sps_lib/Power Grid Elements/Distributed Parameters Line
  LVD7 : spsThreePhaseVIMeasurementLib/Three-Phase V-I Measurement  VoltageMeasurement=no  SetLabelV=on  LabelV=Vabc_LVD7  Vpu=on  VpuLL=off  CurrentMeasurement=no  SetLabelI=off  LabelI=A1  Ipu=off  Pbase=100e6  Vbase=735e3  OutputType=Magnitude  PhasorSimulation=off  PSBequivalent=0
  Load Flow Bus1 : spsLoadFlowBusLib/Load Flow Bus  LConnTagsString=a  Phases=single  Connectors=on one side  ID=LG31_13.8  Vbase=13.8e3  Vref=1  Vangle=0  VLF=1  VLFb=1  VLFc=1  angleLF=-0.0351  angleLFb=0  angleLFc=0
      settings: AttributesFormatString=%<ID>\n%<Vbase>V\n%<VLF>pu\n%<angleLF>deg.
  Load Flow Bus10 : spsLoadFlowBusLib/Load Flow Bus  LConnTagsString=a  Phases=single  Connectors=on one side  ID=LVD7  Vbase=735e3  Vref=1  Vangle=0  VLF=1.05  VLFb=1  VLFc=1  angleLF=-12.02  angleLFb=0  angleLFc=0
      settings: AttributesFormatString=%<ID>\n%<Vbase>V\n%<VLF>pu\n%<angleLF>deg.
  Load Flow Bus11 : spsLoadFlowBusLib/Load Flow Bus  LConnTagsString=a  Phases=single  Connectors=on one side  ID=CHM7  Vbase=735e3  Vref=1  Vangle=0  VLF=1.047  VLFb=1  VLFc=1  angleLF=-4.064  angleLFb=0  angleLFc=0
      settings: AttributesFormatString=%<ID>\n%<Vbase>V\n%<VLF>pu\n%<angleLF>deg.
  Load Flow Bus12 : spsLoadFlowBusLib/Load Flow Bus  LConnTagsString=a  Phases=single  Connectors=on one side  ID=LG47  Vbase=735e3  Vref=1  Vangle=0  VLF=1.004  VLFb=1  VLFc=1  angleLF=20.71  angleLFb=0  angleLFc=0
      settings: AttributesFormatString=%<ID>\n%<Vbase>V\n%<VLF>pu\n%<angleLF>deg.
  Load Flow Bus2 : spsLoadFlowBusLib/Load Flow Bus  LConnTagsString=a  Phases=single  Connectors=on one side  ID=LG3_13.8  Vbase=13.8e3  Vref=1  Vangle=0  VLF=1  VLFb=1  VLFc=1  angleLF=-0.6025  angleLFb=0  angleLFc=0
      settings: AttributesFormatString=%<ID>\n%<Vbase>V\n%<VLF>pu\n%<angleLF>deg.
  Load Flow Bus3 : spsLoadFlowBusLib/Load Flow Bus  LConnTagsString=a  Phases=single  Connectors=on one side  ID=LG4_13.8  Vbase=13.8e3  Vref=1  Vangle=0  VLF=1  VLFb=1  VLFc=1  angleLF=-3.293  angleLFb=0  angleLFc=0
      settings: AttributesFormatString=%<ID>\n%<Vbase>V\n%<VLF>pu\n%<angleLF>deg.
  Load Flow Bus4 : spsLoadFlowBusLib/Load Flow Bus  LConnTagsString=a  Phases=single  Connectors=on one side  ID=LG2_13.8  Vbase=13.8e3  Vref=1  Vangle=0  VLF=1  VLFb=1  VLFc=1  angleLF=0  angleLFb=0  angleLFc=0
      settings: AttributesFormatString=%<ID>\n%<Vbase>V\n%<VLF>pu\n%<angleLF>deg.
  Load Flow Bus5 : spsLoadFlowBusLib/Load Flow Bus  LConnTagsString=a  Phases=single  Connectors=on one side  ID=LG27  Vbase=735e3  Vref=1  Vangle=0  VLF=1  VLFb=1  VLFc=1  angleLF=23.57  angleLFb=0  angleLFc=0
      settings: AttributesFormatString=%<ID>\n%<Vbase>V\n%<VLF>pu\n%<angleLF>deg.
  Load Flow Bus6 : spsLoadFlowBusLib/Load Flow Bus  LConnTagsString=a  Phases=single  Connectors=on one side  ID=LG37  Vbase=735e3  Vref=1  Vangle=0  VLF=0.994  VLFb=1  VLFc=1  angleLF=24.1  angleLFb=0  angleLFc=0
      settings: AttributesFormatString=%<ID>\n%<Vbase>V\n%<VLF>pu\n%<angleLF>deg.
  Load Flow Bus7 : spsLoadFlowBusLib/Load Flow Bus  LConnTagsString=a  Phases=single  Connectors=on one side  ID=LMO7  Vbase=735e3  Vref=1  Vangle=0  VLF=1.016  VLFb=1  VLFc=1  angleLF=17.31  angleLFb=0  angleLFc=0
      settings: AttributesFormatString=%<ID>\n%<Vbase>V\n%<VLF>pu\n%<angleLF>deg.
  Load Flow Bus8 : spsLoadFlowBusLib/Load Flow Bus  LConnTagsString=a  Phases=single  Connectors=on one side  ID=NEM_ALB7  Vbase=735e3  Vref=1  Vangle=0  VLF=1.028  VLFb=1  VLFc=1  angleLF=8.928  angleLFb=0  angleLFc=0
      settings: AttributesFormatString=%<ID>\n%<Vbase>V\n%<VLF>pu\n%<angleLF>deg.
  Load Flow Bus9 : spsLoadFlowBusLib/Load Flow Bus  LConnTagsString=a  Phases=single  Connectors=on one side  ID=ABI_CHB7  Vbase=735e3  Vref=1  Vangle=0  VLF=1.046  VLFb=1  VLFc=1  angleLF=0.1334  angleLFb=0  angleLFc=0
      settings: AttributesFormatString=%<ID>\n%<Vbase>V\n%<VLF>pu\n%<angleLF>deg.
  NEM-ABI 6*236 : spsDistributedParametersLineLib/Distributed Parameters Line  Phases=3  Length=236  Frequency=60  Resistance="[0.01273  0.3864]/6"  Inductance="[0.9337e-3  4.1264e-3]/6"  Capacitance=[12.74e-9 7.751e-9]*6  x1=[-0.00135 1.5807353464931e-08 0 0;-0.001275 1.58478089967828e-08 0 0;-0.0012 1.58755960326022e-08 0 0;-0.001125 1.58906923598578e-08 0 0;-0.00105 1.58930859107768e-08 0 0;-0.000975 1.58827747719911e-08 0 0;-0.0009 1.58597671860672e-08 0 0;-0.000825 1.58240815449173e-08 284117.477880567 -680689.106292036;-0.00075 1.57757463750971e-08 303247.373018711 -672384.845537065;-0.000675 1.57148003150016e-08 322134.856846704 -663543.090624405;-0.0006 1.56412920839787e-08 340764.830998962 -654170.90951765;-0.000525 1.55552804433838e-08 359122.402959197 -644275.794194976;-0.00045 1.54568341496061e-08 377192.897965263 -633865.654660174;-0.000375 1.53460318991068e-08 394961.87073994 -622948.812619505;-0.0003 1.52229622655095e-08 412415.117038268 -611533.994829466;-0.000225 1.50877236287963e-08 429538.685002197 -599630.326120743;-0.00015 1.49404240966641e-08 446318.886313499 -587247.322103971;-7.5e-05 1.47811814181052e-08 462742.307135989 -574394.881563095]  x2=[-0.00135 2.87989522022822e-08 0 0;-0.001275 2.88412839669071e-08 0 0;-0.0012 2.88605604504152e-08 0 0;-0.001125 2.88567662434807e-08 0 0;-0.00105 2.88299043791344e-08 0 0;-0.000975 2.87799963303398e-08 0 0;-0.0009 2.87070819928275e-08 0 0;-0.000825 2.86112196532031e-08 125357.104453994 -735061.346284902;-0.00075 2.84924859423543e-08 146087.597415342 -731223.617196954;-0.000675 2.83509757741929e-08 166701.310186531 -726801.359137515;-0.0006 2.81868022697821e-08 187181.764480972 -721798.107192015;-0.000525 2.80000966669093e-08 207512.588536865 -716217.860883508;-0.00045 2.77910082151768e-08 227677.53020453 -710065.080975511;-0.000375 2.75597040566938e-08 247660.469938132 -703344.685906142;-0.0003 2.73063690924655e-08 267445.433681399 -696062.047856394;-0.000225 2.70312058345862e-08 287016.605637032 -688222.988455697;-0.00015 2.6734434244354e-08 306358.340909621 -679833.774128193;-7.5e-05 2.64162915564374e-08 325455.178011927 -670901.111083456]  x3=[-0.00135 1.59972187215109e-10 0 0;-0.001275 1.66798367029797e-10 0 0;-0.0012 1.73491210781983e-10 0 0;-0.001125 1.80045368314773e-10 0 0;-0.00105 1.8645560033492e-10 0 0;-0.000975 1.92716782601025e-10 0 0;-0.0009 1.98823910019784e-10 0 0;-0.000825 2.04772100646982e-10 -448.18748211001 -4499.57322109539;-0.00075 2.1055659959004e-10 -320.801895602983 -4510.4440485975;-0.000675 2.1617278280901e-10 -193.159864969044 -4517.70929613926;-0.0006 2.21616160812958e-10 -65.3634252944938 -4521.36315599296;-0.000525 2.26882382248792e-10 62.4852649021427 -4521.40270731893;-0.00045 2.31967237379673e-10 190.284005334073 -4517.82791850045;-0.000375 2.36866661450211e-10 317.930635643582 -4510.64164716902;-0.0003 2.41576737935767e-10 445.32311706746 -4499.84963791996;-0.000225 2.46093701673265e-10 572.359614005226 -4485.46051772036;-0.00015 2.50413941871006e-10 698.938575424952 -4467.48578901274;-7.5e-05 2.54534004995076e-10 824.958816041602 -4445.93982052021]  x4=[-0.00135 1.65119599851683e-10 0 0;-0.001275 1.61545483276445e-10 0 0;-0.0012 1.57842229713606e-10 0 0;-0.001125 1.540127994874e-10 0 0;-0.00105 1.50060253785759e-10 0 0;-0.000975 1.4598775221324e-10 0 0;-0.0009 1.4179855026529e-10 0 0;-0.000825 1.37495996725848e-10 4622.22438525034 -28011.6084746955;-0.00075 1.33083530990383e-10 5412.27949589112 -27869.7398149546;-0.000675 1.28564680316491e-10 6198.00811311353 -27705.5925116269;-0.0006 1.23943057004259e-10 6978.78213748303 -27519.2977815552;-0.000525 1.1922235550865e-10 7753.97743019077 -27311.0045458964;-0.00045 1.14406349486211e-10 8522.97431198065 -27080.8793110759;-0.000375 1.09498888778468e-10 9285.15805851141 -26829.1060356855;-0.0003 1.04503896334425e-10 10039.9193917579 -26555.8859834292;-0.000225 9.94253650746156e-11 10786.6549670585 -26261.4375622365;-0.00015 9.42673546992246e-11 11524.7678554198 -25945.99614967;-7.5e-05 8.90339884428259e-11 12253.6680206923 -25609.8139047685]  x5=0.00133467809810995  V1=ones(3,3)  V2=ones(3,3)  I1=ones(3,3)  I2=ones(3,3)  nHarmo=1  Measurements=None  Decoupling=on  VsMag0=[602251.717194494 602251.086049818 602251.913986818]  VrMag0=[608840.309919402 608839.972623147 608840.270927347]  VsAngle0=[10.4755045319383 -109.524439182996 130.475584674534]  VrAngle0=[-2.50190241954691 -122.501888330514 117.498132114124]  IsMag0=[3712.64388956053 3712.61521802411 3712.60597455308]  IrMag0=[23309.611878836 23309.6245706249 23309.6488489229]  IsAngle0=[-17.867898304413 -137.868318490095 102.132274803438]  IrAngle0=[-2.81003503241448 -122.80994811205 117.189981410578]
      settings: AttributesFormatString=\n  LibrarySourceBlock=sps_lib/Power Grid Elements/Distributed Parameters Line
  NEM-ALB 1980 Mvar : spsThreePhaseSeriesRLCLoadLib/Three-Phase Series RLC Load  LConnTagsString=A|B|C  Configuration=Y (grounded)  NominalVoltage=735e3  Vabc=[1e3 1e3 1e3]  Vabcp=[1e3 1e3 1e3]  NominalFrequency=60  UnbalancedPower=off  ActivePower=6600000  InductivePower=1980e6  CapacitivePower=0  Pabc=[10e3 9e3 11e3]  QLabc=[100 90 110]  QCabc=[100 90 110]  Pabcp=[10e3 9e3 11e3]  QLabcp=[100 90 110]  QCabcp=[100 90 110]  Measurements=None  LoadType=constant Z
  NEM-ALB7 : spsThreePhaseVIMeasurementLib/Three-Phase V-I Measurement  VoltageMeasurement=no  SetLabelV=on  LabelV=Vabc_NEM7  Vpu=on  VpuLL=off  CurrentMeasurement=no  SetLabelI=off  LabelI=A1  Ipu=off  Pbase=100e6  Vbase=735e3  OutputType=Magnitude  PhasorSimulation=off  PSBequivalent=0
  Regulators1 : Subsystem
  Regulators2 : Subsystem
  Regulators3 : Subsystem
  Regulators4 : Subsystem
  MTLa : PMIOPort  Side=Right
  MTLb : PMIOPort  Port=2  Side=Right
  MTLc : PMIOPort  Port=3  Side=Right
  CHM7a : PMIOPort  Port=4  Side=Right
  CHM7b : PMIOPort  Port=5  Side=Right
  CHM7c : PMIOPort  Port=6  Side=Right
  wires:
  Regulators2/1(Pm) -> LG3_2200 MVA/1
  Regulators4/2(Vf) -> LG4-2700 MVA/2
  Regulators4/1(Pm) -> LG4-2700 MVA/1
  Regulators3/2(Vf) -> LG31-200 MVA/2
  Regulators3/1(Pm) -> LG31-200 MVA/1
  Regulators2/2(Vf) -> LG3_2200 MVA/2
  LG3_2200 MVA/1 -> Regulators2/1(m)
  Regulators1/1(Pm) -> LG2_5500 MVA/1
  Regulators1/2(Vf) -> LG2_5500 MVA/2
  LG2_5500 MVA/1 -> Regulators1/1(m)
  LG31-200 MVA/1 -> Regulators3/1(m)
  LG4-2700 MVA/1 -> Regulators4/1(m)
  connections:
  LG2-NENI 3*279km/RConn1 -- "Cs NEM "/LConn1
  LG2-NENI 3*279km/RConn2 -- "Cs NEM "/LConn2
  LG2-NENI 3*279km/RConn3 -- "Cs NEM "/LConn3
  CHB-CHM 3*195km/RConn1 -- "Cs  CHMN "/LConn1
  CHB-CHM 3*195km/RConn2 -- "Cs  CHMN "/LConn2
  CHB-CHM 3*195km/RConn3 -- "Cs  CHMN "/LConn3
  Load Flow Bus2/LConn1 -- 2200 MVA 13.8 kV/735 kV/LConn1 -- LG3_2200 MVA/RConn1 -- 110 MW/LConn1
  2200 MVA 13.8 kV/735 kV/LConn2 -- LG3_2200 MVA/RConn2 -- 110 MW/LConn2
  2200 MVA 13.8 kV/735 kV/LConn3 -- LG3_2200 MVA/RConn3 -- 110 MW/LConn3
  Load Flow Bus1/LConn1 -- 200 MVA 13.8 kV/735 kV/LConn1 -- LG31-200 MVA/RConn1 -- 10 MW/LConn1
  200 MVA 13.8 kV/735 kV/LConn2 -- LG31-200 MVA/RConn2 -- 10 MW/LConn2
  200 MVA 13.8 kV/735 kV/LConn3 -- LG31-200 MVA/RConn3 -- 10 MW/LConn3
  Load Flow Bus6/LConn1 -- 2200 MVA 13.8 kV/735 kV/RConn1 -- 200 MVA 13.8 kV/735 kV/RConn1 -- LG3-LMO 104km/LConn1 -- LG3 660 Mvar/LConn1 -- LG2-LG3 155km/RConn1
  2200 MVA 13.8 kV/735 kV/RConn2 -- LG3 660 Mvar/LConn2 -- LG2-LG3 155km/RConn2 -- 200 MVA 13.8 kV/735 kV/RConn2 -- LG3-LMO 104km/LConn2
  LG3-LMO 104km/RConn1 -- LMO7/RConn1 -- LG4-LMO 3*118km/RConn1 -- LMO 330 Mvar/LConn1
  LG3-LMO 104km/RConn2 -- LMO7/RConn2 -- LG4-LMO 3*118km/RConn2 -- LMO 330 Mvar/LConn2
  LG3-LMO 104km/RConn3 -- LMO7/RConn3 -- LG4-LMO 3*118km/RConn3 -- LMO 330 Mvar/LConn3
  LG4-LMO 3*118km/LConn1 -- LG4 660 Mvar/LConn1 -- 2700 MVA 13.8 kV/735 kV/RConn1 -- Load Flow Bus12/LConn1
  LG4-LMO 3*118km/LConn2 -- 2700 MVA 13.8 kV/735 kV/RConn2 -- LG4 660 Mvar/LConn2
  LG4 660 Mvar/LConn3 -- 2700 MVA 13.8 kV/735 kV/RConn3 -- LG4-LMO 3*118km/LConn3
  Load Flow Bus3/LConn1 -- LG4-2700 MVA/RConn1 -- 2700 MVA 13.8 kV/735 kV/LConn1 -- 135 MW/LConn1
  LG4-2700 MVA/RConn2 -- 2700 MVA 13.8 kV/735 kV/LConn2 -- 135 MW/LConn2
  LG4-2700 MVA/RConn3 -- 2700 MVA 13.8 kV/735 kV/LConn3 -- 135 MW/LConn3
  Load Flow Bus4/LConn1 -- 5500 MVA 13.8 kV/735 kV/LConn1 -- LG2_5500 MVA/RConn1 -- 275 MW/LConn1
  5500 MVA 13.8 kV/735 kV/LConn2 -- LG2_5500 MVA/RConn2 -- 275 MW/LConn2
  LG2_5500 MVA/RConn3 -- 5500 MVA 13.8 kV/735 kV/LConn3 -- 275 MW/LConn3
  5500 MVA 13.8 kV/735 kV/RConn1 -- LG2-NENI 3*279km/LConn1 -- LG2-LG3 155km/LConn1 -- LG2 660 Mvar/LConn1 -- Load Flow Bus5/LConn1
  LG2-LG3 155km/LConn2 -- 5500 MVA 13.8 kV/735 kV/RConn2 -- LG2-NENI 3*279km/LConn2 -- LG2 660 Mvar/LConn2
  LG2-LG3 155km/LConn3 -- 5500 MVA 13.8 kV/735 kV/RConn3 -- LG2-NENI 3*279km/LConn3 -- LG2 660 Mvar/LConn3
  "Cs NEM "/RConn1 -- NEM-ALB7/LConn1 -- Cs ALB/RConn1
  "Cs NEM "/RConn2 -- NEM-ALB7/LConn2 -- Cs ALB/RConn2
  "Cs NEM "/RConn3 -- NEM-ALB7/LConn3 -- Cs ALB/RConn3
  LMO7/LConn1 -- LMO-ALB 3*218km/LConn1
  LMO7/LConn2 -- LMO-ALB 3*218km/LConn2
  Load Flow Bus7/LConn1 -- LMO7/LConn3 -- LMO-ALB 3*218km/LConn3
  Cs ALB/LConn1 -- LMO-ALB 3*218km/RConn1
  Cs ALB/LConn2 -- LMO-ALB 3*218km/RConn2
  Cs ALB/LConn3 -- LMO-ALB 3*218km/RConn3
  200 MVA 13.8 kV/735 kV/RConn3 -- LG3-LMO 104km/LConn3 -- LG3 660 Mvar/LConn3 -- LG2-LG3 155km/RConn3 -- 2200 MVA 13.8 kV/735 kV/RConn3
  Load Flow Bus8/LConn1 -- NEM-ABI 6*236/LConn1 -- NEM-ALB7/RConn1 -- NEM-ALB 1980 Mvar/LConn1
  NEM-ALB 1980 Mvar/LConn2 -- NEM-ALB7/RConn2 -- NEM-ABI 6*236/LConn2
  NEM-ALB 1980 Mvar/LConn3 -- NEM-ALB7/RConn3 -- NEM-ABI 6*236/LConn3
  NEM-ABI 6*236/RConn1 -- "Cs ABI+CHB "/LConn1
  NEM-ABI 6*236/RConn2 -- "Cs ABI+CHB "/LConn2
  NEM-ABI 6*236/RConn3 -- "Cs ABI+CHB "/LConn3
  "Cs ABI+CHB "/RConn1 -- ABI-CHB7/LConn1
  "Cs ABI+CHB "/RConn2 -- ABI-CHB7/LConn2
  "Cs ABI+CHB "/RConn3 -- ABI-CHB7/LConn3
  Load Flow Bus9/LConn1 -- ABI+CHB 1320 Mvar/LConn1 -- CHB-CHM 3*195km/LConn1 -- ABI-CHB 3*271km/LConn1 -- ABI-CHB7/RConn1
  ABI-CHB 3*271km/LConn2 -- ABI-CHB7/RConn2 -- ABI+CHB 1320 Mvar/LConn2 -- CHB-CHM 3*195km/LConn2
  ABI-CHB 3*271km/LConn3 -- ABI-CHB7/RConn3 -- ABI+CHB 1320 Mvar/LConn3 -- CHB-CHM 3*195km/LConn3
  ABI-CHB 3*271km/RConn1 -- "Cs LVDN "/LConn1
  ABI-CHB 3*271km/RConn2 -- "Cs LVDN "/LConn2
  ABI-CHB 3*271km/RConn3 -- "Cs LVDN "/LConn3
  "Cs LVDN "/RConn1 -- LVD7/LConn1
  "Cs LVDN "/RConn2 -- LVD7/LConn2
  "Cs LVDN "/RConn3 -- LVD7/LConn3
  "Cs LVDS "/LConn1 -- LVD 990 Mvar/LConn1 -- Load Flow Bus10/LConn1 -- LVD7/RConn1
  "Cs LVDS "/LConn2 -- LVD7/RConn2 -- LVD 990 Mvar/LConn2
  "Cs LVDS "/LConn3 -- LVD7/RConn3 -- LVD 990 Mvar/LConn3
  "Cs LVDS "/RConn1 -- LVD-MTL 3*260km/LConn1
  "Cs LVDS "/RConn2 -- LVD-MTL 3*260km/LConn2
  "Cs LVDS "/RConn3 -- LVD-MTL 3*260km/LConn3
  MTLa/RConn1 -- LVD-MTL 3*260km/RConn1
  MTLb/RConn1 -- LVD-MTL 3*260km/RConn2
  MTLc/RConn1 -- LVD-MTL 3*260km/RConn3
  "Cs  CHMN "/RConn1 -- CHM7/LConn1
  "Cs  CHMN "/RConn2 -- CHM7/LConn2
  "Cs  CHMN "/RConn3 -- CHM7/LConn3
  CHM 1320Mvar/LConn2 -- CHM7/RConn2 -- CHM7b/RConn1
  Load Flow Bus11/LConn1 -- CHM 1320Mvar/LConn3 -- CHM7c/RConn1 -- CHM7/RConn3
  CHM7a/RConn1 -- CHM 1320Mvar/LConn1 -- CHM7/RConn1
